simulink model "sun_point_unit_test"  (R2016b)
settings: Solver=VariableStepAuto  StartTime=0.0  StopTime=1000  MaxStep=0.01  RelTol=1e-4  EnableMultiTasking=on
libraries: aerolibutil x5, sun_point_lib x1
settings Model: Creator=Krish  LastModifiedBy=Krish
settings DataIOCC: LimitDataPoints=on  SaveOutput=off  SaveTime=off
settings OptimizationCC: ExpressionDepthLimit=2147483647  LifeSpan=1
settings DebuggingCC: UnderspecifiedInitializationDetection=Classic  MergeDetectMultiDrivingBlocksExec=none  FcnCallInpInsideContextMsg=warning  AllowSymbolicDim=off  StateNameClashWarn=warning  SFUnexpectedBacktrackingDiag=warning  SFNoUnconditionalDefaultTransitionDiag=warning  SFExecutionAtInitializationDiag=none
settings GRTTargetCC: TargetLangStandard=C89/C90 (ANSI)  GeneratePreprocessorConditionals=Disable all  CombineOutputUpdateFcns=off  GRTInterface=on

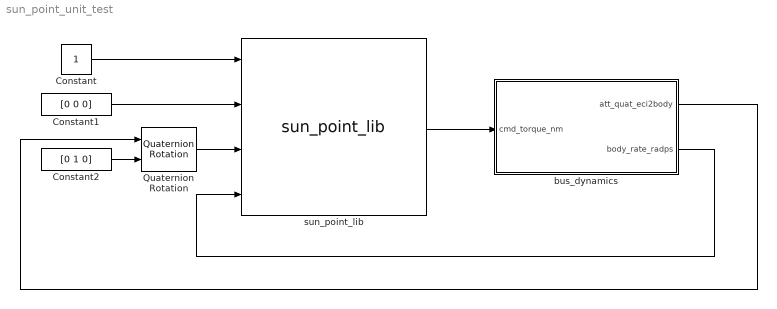
== system sun_point_unit_test ==
  Constant : Constant
  Constant1 : Constant  Value=[0 0 0]
  Constant2 : Constant  Value=[0 1 0]
  Quaternion Rotation : aerolibutil/Quaternion Rotation
  bus_dynamics : Subsystem
  sun_point_lib : sun_point_lib/sun_point_lib
  wires:
  sun_point_lib/1 -> bus_dynamics/1(cmd_torque_nm)
  Constant/1 -> sun_point_lib/1
  Constant1/1 -> sun_point_lib/2
  Quaternion Rotation/1 -> sun_point_lib/3
  Constant2/1 -> Quaternion Rotation/2
  bus_dynamics/1(att_quat_eci2body) -> Quaternion Rotation/1
  bus_dynamics/2(body_rate_radps) -> sun_point_lib/4

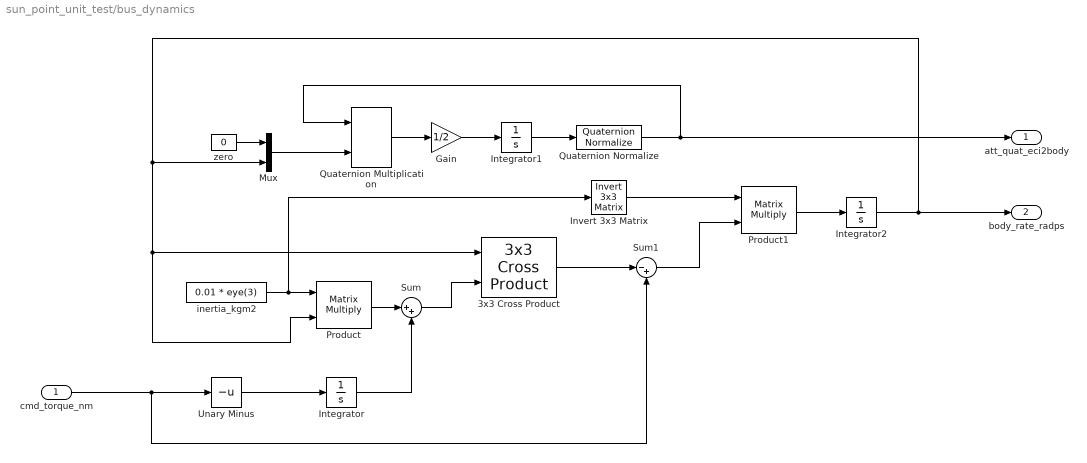
== system sun_point_unit_test/bus_dynamics ==
  cmd_torque_nm : Inport
  3x3 Cross Product : aerolibutil/3x3 Cross Product
  Gain : Gain  Gain=1/2
  Integrator : Integrator  InitialCondition=[0 0 0]
  Integrator1 : Integrator  InitialCondition=[1 0 0 0]
  Integrator2 : Integrator  InitialCondition=[0 0 0]
  Invert 3x3 Matrix : aerolibutil/Invert  3x3 Matrix
  Mux : Mux  Inputs=[1 3]
  Product : Product  Multiplication=Matrix(*)
  Product1 : Product  Multiplication=Matrix(*)
  Quaternion Multiplication : aerolibutil/Quaternion Multiplication
  Quaternion Normalize : aerolibutil/Quaternion Normalize
  Sum : Sum  Inputs=|++
  Sum1 : Sum  Inputs=|-+
  Unary Minus : UnaryMinus
  inertia_kgm2 : Constant  Value=0.01 * eye(3)
  zero : Constant  Value=0
  att_quat_eci2body : Outport
  body_rate_radps : Outport  Port=2
  wires:
  Quaternion Normalize/1 -> att_quat_eci2body/1, Quaternion Multiplication/1
  Integrator2/1 -> body_rate_radps/1, 3x3 Cross Product/1, Product/2, Mux/2
  Product/1 -> Sum/1
  Sum/1 -> 3x3 Cross Product/2
  Integrator/1 -> Sum/2
  3x3 Cross Product/1 -> Sum1/1
  Integrator1/1 -> Quaternion Normalize/1
  zero/1 -> Mux/1
  Mux/1 -> Quaternion Multiplication/2
  Quaternion Multiplication/1 -> Gain/1
  Gain/1 -> Integrator1/1
  inertia_kgm2/1 -> Invert 3x3 Matrix/1, Product/1
  Invert 3x3 Matrix/1 -> Product1/1
  Sum1/1 -> Product1/2
  cmd_torque_nm/1 -> Unary Minus/1, Sum1/2
  Product1/1 -> Integrator2/1
  Unary Minus/1 -> Integrator/1
